simulink model "testSim"  (R2016b)
settings: Solver=VariableStepAuto  StartTime=0.0  StopTime=30  RelTol=1e-4
values from neighbouring files (symbols this model uses):
  A_stab = [A_lon_stab,zeros(4,5);zeros(5,4),A_lat]    [AutoStab.m]    (also in Stab.m)
  B = [2.07005,0,0,9.57054;     -88.0560,0,0,0;     -20.5780,0,0,-0.143558;     0,0,0,0;     0,12.2129,14.4466,0;     0,-84.7711,15.1058,0;     0,-3.25531,-6.83654,0;     0,0,0,0;     0,0,0,0]    [param.m]    (also in paramDYB.m = [2.07005,0,0,9.57054;     -40.0560,0,0,0;     -10.5780,0,0,-)
  C = [ ... (first row only)    [controlmodel.m]    (also in param.m = [-0.0498445,-1.35067,4.39526,0,0,0,0,0,0;     0,0,0,0,-0.095; paramDYB.m = [-0.0498445,-1.35067,4.39526,0,0,0,0,0,0;     0,0,0,0,-0.095; planemodel.m)
  D = [12.0969,0,0,0.698697;     0,-40.4214,-12.2709,0;     0,0,0,0;     0,0,0,0]    [param.m]    (also in paramDYB.m)
  X0 = [0;-17.7459;0;0;0;0;0;0;0]    [param.m]    (also in paramDYB.m = [0;0;0;0;0;0;0;0;0])
undefined symbols (not defined in the file or in its folder): drawplane
settings Model: Creator=CFRPG  LastModifiedBy=CFRPG

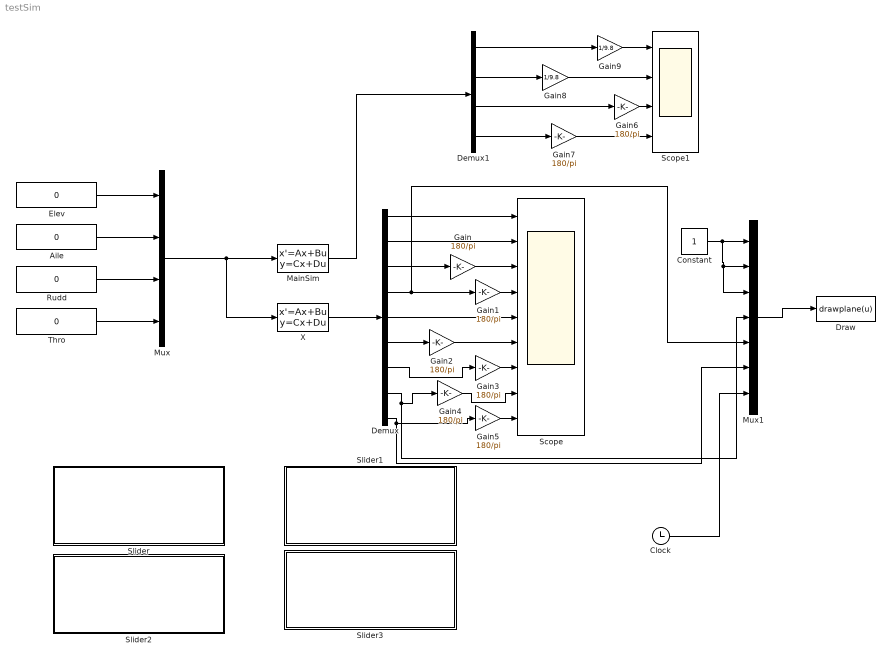
== system testSim ==
  Aile : Constant  Value=0
  Clock : Clock
  Constant : Constant
  Demux : Demux  Outputs=9
  Demux1 : Demux
  Draw : MATLABFcn  MATLABFcn=drawplane(u)  OutputDimensions=0
  Elev : Constant  Value=0
  Gain{,1..7} (8 alike) : Gain  Gain=180/pi
  Gain8 : Gain  Gain=1/9.8
  Gain9 : Gain  Gain=1/9.8
  MainSim : StateSpace  A=A_stab  B=B  C=C  D=D  X0=X0
  Mux : Mux
  Mux1 : Mux  Inputs=7
  Rudd : Constant  Value=0
  Scope : Scope  NumInputPorts=9
  Scope1 : Scope  NumInputPorts=4
  Slider : Subsystem  DialogController=hmiCreateDDGDialog  IsWebBlock=on  mask(MWDashboardBlock){webBlockId=e457a40e-dc7d-44c2-be31-dd759c580c2b, webBlockType=slider, ShowInLibBrowser=on, ShowInitialText=on, HMISrcModelName=testSim}
      mask prompts: webBlockId "WebBlock Id"; webBlockType "WebBlock Type"; HMISrcModelName "Source Model"
      mask help: SimulinkHMI:dialogs:SliderDialogDesc
      mask Help: helpview([docroot '/mapfiles/simulink.map'], 'hmi_slider')
      mask Display:
      | if strcmp(get_param(bdroot(gcb),'BlockDiagramType'), 'library')
      |     image([(matlabroot) '/toolbox/simulink/hmi/icons/Slider.png']);
      | end
  Slider1 : Subsystem  DialogController=hmiCreateDDGDialog  IsWebBlock=on  mask(MWDashboardBlock){webBlockId=4ed8795a-3806-45b2-8487-915766386259, webBlockType=slider, ShowInLibBrowser=on, ShowInitialText=on, HMISrcModelName=testSim}
      mask prompts: webBlockId "WebBlock Id"; webBlockType "WebBlock Type"; HMISrcModelName "Source Model"
      mask help: SimulinkHMI:dialogs:SliderDialogDesc
      mask Help: helpview([docroot '/mapfiles/simulink.map'], 'hmi_slider')
      mask Display:
      | if strcmp(get_param(bdroot(gcb),'BlockDiagramType'), 'library')
      |     image([(matlabroot) '/toolbox/simulink/hmi/icons/Slider.png']);
      | end
  Slider2 : Subsystem  DialogController=hmiCreateDDGDialog  IsWebBlock=on  mask(MWDashboardBlock){webBlockId=9539b736-92d7-47d4-86f8-32d613f5a1b0, webBlockType=slider, ShowInLibBrowser=on, ShowInitialText=on, HMISrcModelName=testSim}
      mask prompts: webBlockId "WebBlock Id"; webBlockType "WebBlock Type"; HMISrcModelName "Source Model"
      mask help: SimulinkHMI:dialogs:SliderDialogDesc
      mask Help: helpview([docroot '/mapfiles/simulink.map'], 'hmi_slider')
      mask Display:
      | if strcmp(get_param(bdroot(gcb),'BlockDiagramType'), 'library')
      |     image([(matlabroot) '/toolbox/simulink/hmi/icons/Slider.png']);
      | end
  Slider3 : Subsystem  DialogController=hmiCreateDDGDialog  IsWebBlock=on  mask(MWDashboardBlock){webBlockId=e8be421a-2db6-47db-99ac-e2ad2b5fd6df, webBlockType=slider, ShowInLibBrowser=on, ShowInitialText=on, HMISrcModelName=testSim}
      mask prompts: webBlockId "WebBlock Id"; webBlockType "WebBlock Type"; HMISrcModelName "Source Model"
      mask help: SimulinkHMI:dialogs:SliderDialogDesc
      mask Help: helpview([docroot '/mapfiles/simulink.map'], 'hmi_slider')
      mask Display:
      | if strcmp(get_param(bdroot(gcb),'BlockDiagramType'), 'library')
      |     image([(matlabroot) '/toolbox/simulink/hmi/icons/Slider.png']);
      | end
  Thro : Constant  Value=0
  X : StateSpace  A=A_stab  B=B  C=eye(9)  D=zeros(9,4)  X0=X0
  wires:
  X/1 -> Demux/1
  Demux/2 -> Scope/2
  Demux/3 -> Gain/1
  Demux/4 -> Gain1/1, Mux1/5
  Demux/5 -> Scope/5
  Demux/6 -> Gain2/1
  Demux/7 -> Gain3/1
  Demux/8 -> Gain4/1, Mux1/4
  Demux/9 -> Gain5/1, Mux1/6
  Mux/1 -> X/1, MainSim/1
  Elev/1 -> Mux/1
  Aile/1 -> Mux/2
  Rudd/1 -> Mux/3
  Thro/1 -> Mux/4
  Demux/1 -> Scope/1
  Mux1/1 -> Draw/1
  Constant/1 -> Mux1/3, Mux1/2, Mux1/1
  Clock/1 -> Mux1/7
  Demux1/1 -> Gain9/1
  Demux1/2 -> Gain8/1
  Demux1/3 -> Gain6/1
  Demux1/4 -> Gain7/1
  MainSim/1 -> Demux1/1
  Gain/1 -> Scope/3
  Gain1/1 -> Scope/4
  Gain2/1 -> Scope/6
  Gain3/1 -> Scope/7
  Gain4/1 -> Scope/8
  Gain5/1 -> Scope/9
  Gain6/1 -> Scope1/3
  Gain7/1 -> Scope1/4
  Gain8/1 -> Scope1/2
  Gain9/1 -> Scope1/1

== system testSim/Slider ==

== system testSim/Slider1 ==

== system testSim/Slider2 ==

== system testSim/Slider3 ==
